simulink model "joystick"  (R2019b)
settings: Solver=FixedStepAuto  StartTime=0.0  StopTime=inf  FixedStep=0.01  RelTol=1e-3
libraries: robotlib x1, dspnetwork x1
settings Model: SimulationMode=external  SILPILModeSetting=veronly  ExtModeTrigDuration=2  Creator=ONLY-GOD  LastModifiedBy=ONLY-GOD
settings OptimizationCC: DefaultParameterBehavior=Inlined  EnhancedBackFolding=on  PassReuseOutputArgsAs=Individual arguments  ZeroExternalMemoryAtStartup=off  ZeroInternalMemoryAtStartup=off  MaxStackSize=64  OptimizeBlockOrder=speed  DifferentSizesBufferReuse=on  OptimizationCustomize=off  EfficientTunableParamExpr=on
settings DebuggingCC: ParameterTunabilityLossMsg=error
settings HardwareCC: ProdBitPerPointer=32  ProdBitPerSizeT=32  ProdBitPerPtrDiffT=32  ProdLargestAtomicFloat=None  ProdIntDivRoundTo=Undefined  ProdEndianess=Unspecified  ProdWordSize=32  ProdHWDeviceType=Generic->Unspecified (assume 32-bit Generic)
settings SFSimCC: MATLABDynamicMemAlloc=off
settings RTWCC: SystemTargetFile=ert.tlc  TemplateMakefile=ert_default_tmf  GenerateReport=on  Toolchain=Catkin  BuildConfiguration=Faster Runs  IncludeHyperlinkInReport=on  LaunchReport=on  GenerateTraceInfo=on  GenerateTraceReport=on  GenerateTraceReportSl=on  GenerateTraceReportSf=on  GenerateTraceReportEml=on
settings CodeAppCC: ForceParamTrailComments=on  IgnoreCustomStorageClasses=off  OperatorAnnotations=on  SimulinkDataObjDesc=on  SFDataObjDesc=on  InsertBlockDesc=on
settings ERTTargetCC: SupportContinuousTime=on  ExtModeStaticAllocSize=250  ERTCustomFileTemplate=example_file_process.tlc

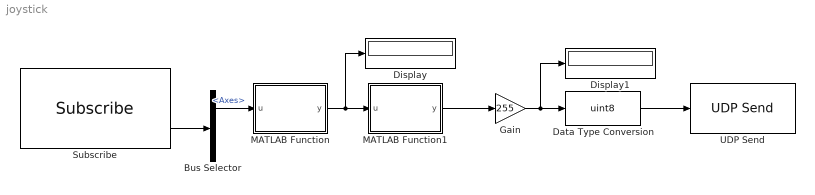
== system joystick ==
  Bus Selector : BusSelector  OutputSignals=Axes,Buttons
  Data Type Conversion : DataTypeConversion  OutDataTypeStr=uint8
  Display : Display
  Display1 : Display
  Gain : Gain  Gain=255
  MATLAB Function : MATLAB Function  TreatAsAtomicUnit=on
  MATLAB Function1 : MATLAB Function  TreatAsAtomicUnit=on
  Subscribe : robotlib/Subscribe  topicSource=Select from ROS network  topic=/joy  messageType=sensor_msgs/Joy  sampleTime=-1  messageQueueLength=1
      settings: SourceProductName=ROS Toolbox
  UDP Send : dspnetwork/UDP Send  remoteURL='192.168.0.120'  remotePort=56789  localURL='0.0.0.0'  localPortSource=Automatically determine  localPort=-1  sampletime=-1  blockPlatform=[]  separateLengthPort=0
      settings: SourceProductName=Simulink
  wires:
  MATLAB Function1/1(y) -> Gain/1
  Bus Selector/1 -> MATLAB Function/1(u)  "<Axes>"
  Subscribe/2 -> Bus Selector/1
  Data Type Conversion/1 -> UDP Send/1
  Gain/1 -> Display1/1, Data Type Conversion/1
  MATLAB Function/1(y) -> Display/1, MATLAB Function1/1(u)

== matlab function joystick/MATLAB Function1 ==
  data: u input; y output
function y = fcn(u)
y=(sign(u)+1)/2;

== matlab function joystick/MATLAB Function ==
  data: u input; y output
function y = fcn(u)

y = u(1);
